simulink library "InputMixerBtc"  (R2022b)
settings: Solver=VariableStepAuto  StartTime=0.0  StopTime=10.0  RelTol=1e-3
libraries: TuneVar x2, FeaturePath x1, HandyTextFile x1, RTC x1
settings Model: Creator=kl13806  LastModifiedBy=kl13806
settings SolverCC: AlgebraicLoopSolver=TrustRegion
settings DebuggingCC: UnconnectedInputMsg=warning  UnconnectedOutputMsg=warning  UnconnectedLineMsg=warning  SFMachineParentedDataDiag=warning
settings ModelReferenceCC: EnableRefExpFcnMdlSchedulingChecks=on
settings RTWCC: DLArmComputeVersion=19.05

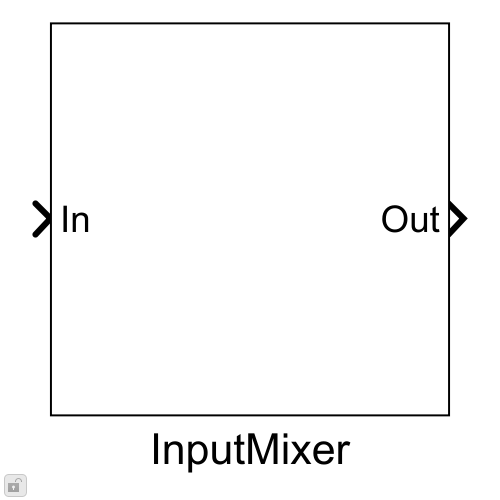
[thumbnail: Simulink's stored preview of the top-level diagram]
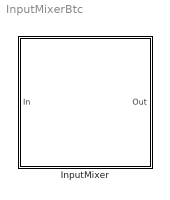
== system InputMixerBtc ==
  InputMixer : Subsystem  mask(Blocklib InputMixer){Config=[], FeatureName=Mixer}
      mask prompts: Config "InputMixerConfig"; FeatureName "Feature path name:"
      mask help:
      | This block will mix N input channels to M output channels (set at build-time), with the type specified.
      |
      | Choose 1 of the 10 types of mixing types, as follows (Type 8 is default):
      | 1: (C) to (L, R)
      | 2: (C, LFE) to (L, R)
      | 3: (L, R) to (L, R)
      | 4: (L, R, C) to (L, R)
      | 5: (L, R, LFE) to (L, R)
      | 6: (L, R, C, LFE) to (L, R)
      | 7: (L, R, Ls) to (L, R, Ls, Rs)
      | 8: (L, R, Ls, Rs) to (L, R, Ls, Rs)
      | 9: (L, R, Ls, Rs, Lrs) to (L, R, Ls, Rs)
      | 10: (L, R, Ls, Rs, Lrs, Rrs) to (L, R, Ls, Rs)
      |
      | The RTC accepts these same values (as an override to the tuning) ... plus a value of "0" which indicates that the value specified in the Tuning is active and will be used.
      mask init:
      | blkh=gcbh;
      | Config=BTConfig.Assert(blkh,Config);
      | Config.Validate();
      | BTConfig.InitSetFeatureIfPresent(blkh,'FeatureName');
      mask Callback Config: BTConfig.CallbackHideIfPresent(gcbh,{'FeatureName'});
      mask TypeOptions FeatureName: FeaturePath/FeatureName

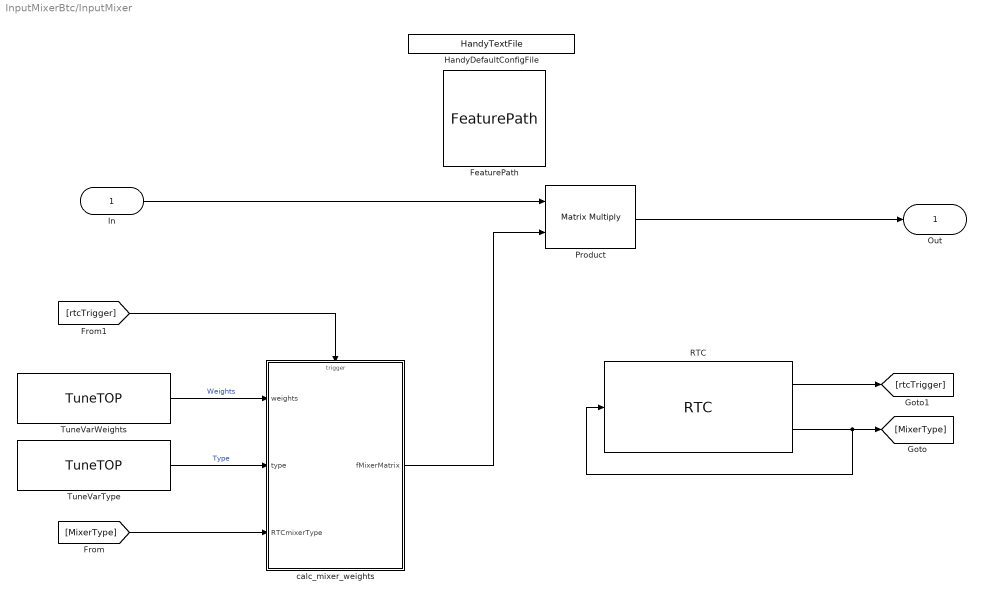
== system InputMixerBtc/InputMixer ==
  In : Inport
  FeaturePath : FeaturePath/FeaturePath  FeatureName=Mixer  IsGroup=off  GroupNumber=-1  IsModule=off  TriggerInit=[420 69 535 176]
      settings: SourceProductName=Bose Talaria
  HandyDefaultConfigFile : HandyTextFile/HandyTextFile  TemplateSource=Config  FileSuffix=Init  OpenDialogOnLoad=off  UseThisBlockName=off  AddGrandParentNamePrefix=off  TheDefaultText=|  ShowInLibBrowser=on
      | % $(FILENAME) Setup model parameters for each "Init" callback (e.g. update diagram)
      | sample_rate_in_hertz = 44100;
      | frame_size = 32;
      | sysin_channel_count = 2;
      settings: SourceProductName=Bose Talaria
  Product : Product  Multiplication=Matrix(*)
  RTC : RTC/RTC  Description=|  REQ_Priority=RTC_Mask.NormalPriority  RequestAtInit=on  EnableRequest=on  REQElemName1=type_index  REQElemType1=uint32  REQElemWidth1=1  REQElemInitial1=0  REQElemType2=uint32  REQElemWidth2=1  REQElemInitial2=[]  REQElemType3=uint32  REQElemWidth3=1  REQElemInitial3=[]  REQElemType4=uint32  REQElemWidth4=1  REQElemInitial4=[]  REQElemType5=uint32  REQElemWidth5=1  REQElemInitial5=[]  REQElemType6=uint32  REQElemWidth6=1  REQElemInitial6=[]  REQElemType7=uint32  REQElemWidth7=1  REQElemInitial7=[]  REQElemType8=uint32  REQElemWidth8=1  REQElemInitial8=[]  REQElemType9=uint32  REQElemWidth9=1  REQElemInitial9=[]  REQElemType10=uint32  REQElemWidth10=1  REQElemInitial10=[]  EnableResponse=on  EnableRSP_StatusIn=off  RSPElemName1=type_index  RSPElemType1=uint32  RSPElemWidth1=1  RSPElemType2=uint32  RSPElemWidth2=1  RSPElemType3=uint32  RSPElemWidth3=1  RSPElemType4=uint32  RSPElemWidth4=1  RSPElemType5=uint32  RSPElemWidth5=1  RSPElemType6=uint32  RSPElemWidth6=1  RSPElemType7=uint32  RSPElemWidth7=1  RSPElemType8=uint32  RSPElemWidth8=1  RSPElemType9=uint32  RSPElemWidth9=1  RSPElemType10=uint32  RSPElemWidth10=1  EnableNotification=off  EnableNTF_PrepTrig=off  NTFElemType1=uint32  NTFElemWidth1=1  NTFElemType2=uint32  NTFElemWidth2=1  NTFElemType3=uint32  NTFElemWidth3=1  NTFElemType4=uint32  NTFElemWidth4=1  NTFElemType5=uint32  NTFElemWidth5=1  NTFElemType6=uint32  NTFElemWidth6=1  NTFElemType7=uint32  NTFElemWidth7=1  NTFElemType8=uint32  NTFElemWidth8=1  NTFElemType9=uint32  NTFElemWidth9=1  NTFElemType10=uint32  NTFElemWidth10=1  MaskMessageName=SetType
      | 0: DEFER to Tuning to determine mixer type
      |  1: (C) to (L, R)
      |  2: (C, LFE) to (L, R)
      |  3: (L, R) to (L, R)
      |  4: (L, R, C) to (L, R)
      |  5: (L, R, LFE) to (L, R)
      |  6: (L, R, C, LFE) to (L, R)
      |  7: (L, R, Ls) to (L, R, Ls, Rs)
      |  8: (L, R, Ls, Rs) to (L, R, Ls, Rs)
      |  9: (L, R, Ls, Rs, Lrs) to (L, R, Ls, Rs)
      |  10: (L, R, Ls, Rs, Lrs, Rrs) to (L, R, Ls, Rs) 
      | 
      | Tuning default might be 8 (depends on tuning of course)
      settings: SourceProductName=Bose Talaria
  TuneVarType : TuneVar/TuneTOP  TriggerInit=[-55 482 115 538]  TopName=Type  TuneName=Type  DataType=single  TunabilityNumber=1  MinValue=[]  MaxValue=[]  BankNumber=0  PreOverlay=false  PostOverlay=false  UseSameName=on  MaskValue=Config.DefaultMixerType
      settings: SourceProductName=Bose Talaria
  TuneVarWeights : TuneVar/TuneTOP  TriggerInit=[-55 407 115 463]  TopName=Weights  TuneName=Weights  DataType=single  TunabilityNumber=1  MinValue=[]  MaxValue=[]  BankNumber=0  PreOverlay=false  PostOverlay=false  UseSameName=on  MaskValue=Config.DefaultWeights
      settings: SourceProductName=Bose Talaria
  calc_mixer_weights : MATLAB Function  TreatAsAtomicUnit=on  mask{MaskNumInputChans=Config.NumInputChans, MaskNumOutputChans=Config.NumOutputChans}
  Out : Outport  VectorParamsAs1DForOutWhenUnconnected=off
  wires:
  calc_mixer_weights/1(fMixerMatrix) -> Product/2
  RTC/1 -> [rtcTrigger]
  [rtcTrigger] -> calc_mixer_weights/Trigger
  [MixerType] -> calc_mixer_weights/3(RTCmixerType)
  RTC/2 -> [MixerType], RTC/1
  TuneVarType/1 -> calc_mixer_weights/2(type)  "Type"
  TuneVarWeights/1 -> calc_mixer_weights/1(weights)  "Weights"
  Product/1 -> Out/1
  In/1 -> Product/1

== matlab function InputMixerBtc/InputMixer/calc_mixer_weights ==
  data: weights input; fMixerMatrix output; type input; RTCmixerType input; MaskNumInputChans parameter; MaskNumOutputChans parameter
  events: trigger input FUNCTION_CALL_EVENT
function fMixerMatrix = fcn(weights, type, RTCmixerType, MaskNumInputChans, MaskNumOutputChans)

%     DESCRIPTION: The matrix "weights" describes 10 different types of
%     mixer weights that can be applied to an incoming audio signal. Each
%     type will mix an incoming signal differently, depending on the
%     associated weights. For instance, in the case of Type 8, we see a
%     value of 1.0 for the columns L2L/R2R, Ls2LS, and Rs2Rs. This means
%     that we will be passing the incoming Left and Right content
%     unaffected, because they will be multiplied by a factor of 1.0.
%     Similarly, we will be passing Left Surround and Right Surround
%     unaffected. In all cases (where the input is 5.1) we always pass
%     Center (C) and Bass (Lfe) content unaffected.
%     In the case of Type 10, we will pass Left to Left and Right to Right
%     unaffected, and then, we see a coefficient of 0.5 for Ls2Ls, Rs2Rs,
%     Lrs2Ls, and Rrs2Rs. This means that the output channels Ls and Rs
%     will be computed by a combination of the input signals Ls, Rs, Lrs,
%     and Rrs:
%               TYPE 10
%           L(out) = L(in)
%           R(out) = R(in)
%           C(out) = C(in)
%           Lfe(out) = Lfe(in)
%           Ls(out) = 0.5 * Ls(in) + 0.5 * Lrs(in)
%           Rs(out) = 0.5 * Rs(in) + 0.5 * Rrs(in)
    
    % Incoming channel description:
    %        If nIn==2: L, R
    %        If nIn==6: L, R, Ls, Rs, C, LFE
    %        If nIn==8: L, R, Ls, Rs, C, LFE, Lrs, Rrs

    % weights =[
    % %L2L/R  ,C2L/R,  LFE2L/R,  Ls2Ls,  Rs2Rs,  Rs2Ls,  Ls2Rs,  Lrs2Ls,  Rrs2Rs,  Rrs2Ls,  Lrs2Rs  
    %     % BI_INPUT_MIXER_1:  (C) to (L, R)
    %     0    ,0.5  ,0    ,0    ,0    ,0    ,0    ,0    ,0    ,0    ,0   ... 
    %     % BI_INPUT_MIXER_2:  (C, LFE) to (L, R)
    %     0    ,0.5  ,0.5  ,0    ,0    ,0    ,0    ,0    ,0    ,0    ,0    ...
    %     % BI_INPUT_MIXER_3:  (L, R) to (L, R)
    %     1.0  ,0    ,0    ,0    ,0    ,0    ,0    ,0    ,0    ,0    ,0   ...
    %     % BI_INPUT_MIXER_4:  (L, R, C) to (L, R) 
    %     0.66666666,0.33333333, 0   ,0   ,0   ,0   ,0   ,0   ,0   ,0   ,0 ...
    %     % BI_INPUT_MIXER_5:  (L, R, LFE) to (L, R)
    %     0.66666666,0   ,0.33333333,0   ,0   ,0   ,0   ,0   ,0   ,0   ,0 ...
    %     % BI_INPUT_MIXER_6:  (L, R, C, LFE) to (L, R)
    %     0.5  ,0.25 ,0.25 ,0    ,0    ,0    ,0    ,0    ,0     ,0    ,0 ...
    %     % BI_INPUT_MIXER_7:  (L, R, Ls) to (L, R, Ls, Rs)
    %     1.0  ,0    ,0    ,0.5  ,0    ,0    ,0.5  ,0    ,0     ,0    ,0 ...
    %     % BI_INPUT_MIXER_8:  (L, R, Ls, Rs) to (L, R, Ls, Rs)
    %     1.0  ,0    ,0    ,1.0  ,1.0  ,0    ,0    ,0    ,0     ,0    ,0  ...
    %     % BI_INPUT_MIXER_9:  (L, R, Ls, Rs, Lrs) to (L, R, Ls, Rs)
    %     1.0  ,0    ,0    ,0.5  ,0.5  ,0    ,0    ,0.5  ,0     ,0    ,0.5 ...
    %     % BI_INPUT_MIXER_10: (L, R, Ls, Rs, Lrs, Rrs) to (L, R, Ls, Rs)
    %     1.0  ,0    ,0    ,0.5  ,0.5  ,0    ,0    ,0.5  ,0.5   ,0    , 0 ];

    default_mixer_type = type;

    if RTCmixerType == 0
        input_mixer_type  = default_mixer_type;
    else
        input_mixer_type = single(RTCmixerType);
    end

    index = ((input_mixer_type -1) * size(weights,2)) + 1;
    weights = reshape(weights',1,numel(weights));
    InMixCoeffs = double(weights(index:index+10));

    INMIX_L2L_R2R     = 1.0;
    INMIX_LFE2L_LFE2R = 0; 
    INMIX_C2L_C2R     = 0; 
    INMIX_Rs2Rs       = 1.0; 
    INMIX_Ls2Rs       = 0; 
    INMIX_Ls2Ls       = 1.0; 
    INMIX_Rs2Ls       = 0; 
    INMIX_Rrs2Rs      = 1.0; 
    INMIX_Lrs2Rs      = 0; 
    INMIX_Lrs2Ls      = 1.0; 
    INMIX_Rrs2Ls      = 0; 

    if(MaskNumInputChans > 2)
        INMIX_LFE2L_LFE2R = InMixCoeffs(3);
        INMIX_C2L_C2R     = InMixCoeffs(2);

        INMIX_Rs2Rs       = InMixCoeffs(5);
        INMIX_Ls2Rs       = InMixCoeffs(7);
        INMIX_Ls2Ls       = InMixCoeffs(4);
        INMIX_Rs2Ls       = InMixCoeffs(6);

    end

    if (MaskNumInputChans > 6)
        INMIX_Rrs2Rs       = InMixCoeffs(9);
        INMIX_Lrs2Rs       = InMixCoeffs(11);
        INMIX_Lrs2Ls       = InMixCoeffs(8);
        INMIX_Rrs2Ls       = InMixCoeffs(10);
    else
        INMIX_Rrs2Rs       = 0;
        INMIX_Lrs2Rs       = 0;
        INMIX_Lrs2Ls       = 0;
        INMIX_Rrs2Ls       = 0;
    end

    MixerMatrix = ...
    ... %  L              R              Ls           Rs           C              BASS               Lrs           Rrs            OUTPUTS
          [INMIX_L2L_R2R  0              0            0            INMIX_C2L_C2R  INMIX_LFE2L_LFE2R  0             0;              %L
           0              INMIX_L2L_R2R  0            0            INMIX_C2L_C2R  INMIX_LFE2L_LFE2R  0             0;              %R
           0              0              INMIX_Ls2Ls  INMIX_Rs2Ls  0              0                  INMIX_Lrs2Ls  INMIX_Rrs2Ls;   %Ls
           0              0              INMIX_Ls2Rs  INMIX_Rs2Rs  0              0                  INMIX_Lrs2Rs  INMIX_Rrs2Rs;   %Rs
           0              0              0            0            1.0            0                  0             0;              %C
           0              0              0            0            0              1.0                0             0];             %Bass     
    
   fMixerMatrix = single(MixerMatrix(1:MaskNumOutputChans,1:MaskNumInputChans)');
